simulink model "sk_R3GDL"  (Simulink 9.0)
settings: Solver=ode45  StartTime=0.0  StopTime=30  MaxStep=1e-3  RelTol=1e-3  EnableMultiTasking=on
values from neighbouring files (symbols this model uses):
  A_a = [0.1  0.1  0.1]    [excitacion.m]
  A_b = [0.5  0.5  0.5]    [excitacion.m]
  Icc = [0  2   1]    [excitacion.m]
  tau = 7    [excitacion.m]
  w_a = [2.5  2.5   2.5]    [excitacion.m]
  w_b = [0.5  1 1]    [excitacion.m]
settings Model: Creator=mortega  LastModifiedBy=Raúl  ExtModeTrigMode=oneshot  ExtModeArmWhenConnect=off
settings DataIOCC: SignalLoggingSaveFormat=ModelDataLogs
settings OptimizationCC: BlockReduction=off  BooleanDataType=off  ExpressionDepthLimit=2147483647  InitFltsAndDblsToZero=on
settings DebuggingCC: SaveWithParameterizedLinksMsg=none  SignalResolutionControl=TryResolveAllWithWarning  MultiTaskDSMMsg=warning  MultiTaskCondExecSysMsg=none  FcnCallInpInsideContextMsg=warning  StateNameClashWarn=warning  StrictBusMsg=None
settings HardwareCC: TargetUnknown=on
settings GRTTargetCC: TargetFcnLib=ansi_tfl_tmw.mat  CombineOutputUpdateFcns=off  GRTInterface=on

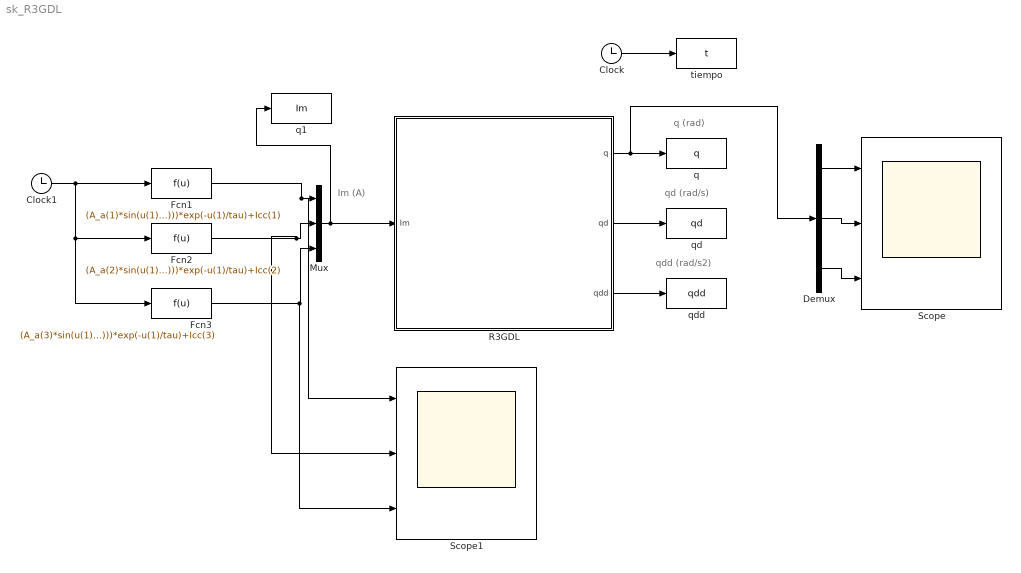
== system sk_R3GDL ==
  note: Im (A)
  note: q (rad)
  note: qd (rad/s)
  note: qdd (rad/s2)
  Clock : Clock
  Clock1 : Clock
  Demux : Demux  Outputs=3
  Fcn1 : Fcn  Expr=(A_a(1)*sin(u(1)*2*pi*w_a(1)) +A_b(1)*sin(u(1)*2*pi*w_b(1)))*exp(-u(1)/tau)+Icc(1)
  Fcn2 : Fcn  Expr=(A_a(2)*sin(u(1)*2*pi*w_a(2)) +A_b(2)*sin(u(1)*2*pi*w_b(2)))*exp(-u(1)/tau)+Icc(2)
  Fcn3 : Fcn  Expr=(A_a(3)*sin(u(1)*2*pi*w_a(3)) +A_b(3)*sin(u(1)*2*pi*w_b(3)))*exp(-u(1)/tau)+Icc(3)
  Mux : Mux  Inputs=3
  R3GDL : Subsystem  mask(Control y Programación de Robots (4 GIERM)){NGrupo=3, q1_ini=0, q2_ini=0, q3_ini=0, Bl_q1=off, Bl_q2=off, Bl_q3=off, AccionamientoDirecto=off}
      mask prompts: NGrupo "Nº de GRUPO"; q1_ini "q1 inicial  (rad)"; q2_ini "q2 inicial (rad)"; q3_ini "q3_inicial (rad)"; Bl_q1 "Bloqueo q1"; Bl_q2 "Bloqueo q2"; Bl_q3 "Bloqueo q3"; AccionamientoDirecto "Accionamiento directo"
      mask help: Robot de 3 grados de libertad RRR
      mask Display:
      | image(imread('R3GDL_RRR.JPG'));
      | port_label('output', 1, 'q');
      | port_label('output', 2, 'qd');
      | port_label('output', 3, 'qdd');
      | port_label('input', 1, 'Im')
  Scope : Scope  NumInputPorts=3
  Scope1 : Scope  NumInputPorts=3
  q : ToWorkspace  VariableName=q  SampleTime=-1
  q1 : ToWorkspace  VariableName=Im  SampleTime=-1
  qd : ToWorkspace  VariableName=qd  SampleTime=-1
  qdd : ToWorkspace  VariableName=qdd  SampleTime=-1
  tiempo : ToWorkspace  VariableName=t  SampleTime=-1
  wires:
  Clock/1 -> tiempo/1
  R3GDL/1(q) -> Demux/1, q/1
  R3GDL/2(qd) -> qd/1
  R3GDL/3(qdd) -> qdd/1
  Demux/1 -> Scope/1
  Demux/2 -> Scope/2
  Demux/3 -> Scope/3
  Clock1/1 -> Fcn3/1, Fcn2/1, Fcn1/1
  Mux/1 -> R3GDL/1(Im), q1/1
  Fcn1/1 -> Scope1/1, Mux/1
  Fcn2/1 -> Scope1/2, Mux/2
  Fcn3/1 -> Scope1/3, Mux/3

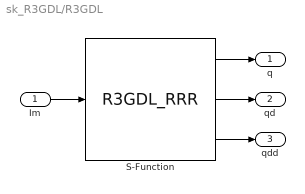
== system sk_R3GDL/R3GDL ==
  Im : Inport
  S-Function : S-Function  FunctionName=R3GDL_RRR  Parameters=[q1_ini; q2_ini; q3_ini]; [Bl_q1; Bl_q2; Bl_q3]; AccionamientoDirecto; NGrupo  SFunctionDeploymentMode=off  EnableBusSupport=off
  q : Outport
  qd : Outport  Port=2
  qdd : Outport  Port=3
  wires:
  Im/1 -> S-Function/1
  S-Function/1 -> q/1
  S-Function/2 -> qd/1
  S-Function/3 -> qdd/1
